simulink model "soar_unit_test"  (R2018b)
settings: Solver=FixedStepAuto  StartTime=0.0  StopTime=600  RelTol=1e-3
values from neighbouring files (symbols this model uses):
  hw0 = Jw * 0.10471975511966 * [ 1000; 1000; 1000 ]    [soar_unit_test_init.m]
  q0 = [ cosd(60/2); sind(60/2).*n ]    [soar_unit_test_init.m]
  qf = [ 1.0; 0.0; 0.0; 0.0 ]    [soar_unit_test_init.m]
  sI = [ 1.0; 0.0; 0.0 ]    [soar_unit_test_init.m]
  w0 = [ 0.0; 0.0; 0.0 ]    [soar_unit_test_init.m]
  wf = [ 0.0; 0.0; 0.0 ]    [soar_unit_test_init.m]
libraries: simulink x2, soar_lib x1
settings Model: Creator=Taylor  LastModifiedBy=Taylor
settings OptimizationCC: DefaultParameterBehavior=Inlined  UseDivisionForNetSlopeComputation=on  UseFloatMulNetSlope=on  InlineInvariantSignals=on  PassReuseOutputArgsAs=Individual arguments  ZeroExternalMemoryAtStartup=off  ZeroInternalMemoryAtStartup=off  NoFixptDivByZeroProtection=on  EfficientFloat2IntCast=on  LifeSpan=1
settings DebuggingCC: ParameterTunabilityLossMsg=error
settings HardwareCC: ProdBitPerPointer=32  ProdBitPerSizeT=32  ProdBitPerPtrDiffT=32  ProdLargestAtomicInteger=Long  ProdWordSize=32  ProdHWDeviceType=ARM Compatible->ARM 7
settings SFSimCC: SimUseLocalCustomCode=off  MATLABDynamicMemAlloc=off
settings RTWCC: SystemTargetFile=ert.tlc  TemplateMakefile=ert_default_tmf  GenerateReport=on  RTWUseLocalCustomCode=off  CustomInclude="\"/Users/Taylor/uw_cubesat_adcs/adcs/sw/components/adcs_oac/include/ecos/include\""  IncludeHyperlinkInReport=on  LaunchReport=on  GenerateTraceInfo=on  GenerateTraceReport=on  GenerateTraceReportSl=on  GenerateTraceReportSf=on  GenerateTraceReportEml=on  GenerateCodeMetricsReport=on
settings RTWCC: CustomSource=|
  | "/Users/Taylor/uw_cubesat_adcs/adcs/sw/components/adcs_oac/include/ecos/src/amd_1.c"
  | "/Users/Taylor/uw_cubesat_adcs/adcs/sw/components/adcs_oac/include/ecos/src/amd_2.c"
  | "/Users/Taylor/uw_cubesat_adcs/adcs/sw/components/adcs_oac/include/ecos/src/amd_aat.c"
  | "/Users/Taylor/uw_cubesat_adcs/adcs/sw/components/adcs_oac/include/ecos/src/amd_control.c"
  | "/Users/Taylor/uw_cubesat_adcs/adcs/sw/components/adcs_oac/include/ecos/src/amd_defaults.c"
  | "/Users/Taylor/uw_cubesat_adcs/adcs/sw/components/adcs_oac/include/ecos/src/amd_dump"
  | "/Users/Taylor/uw_cubesat_adcs/adcs/sw/components/adcs_oac/include/ecos/src/amd_global.c"
  | "/Users/Taylor/uw_cubesat_adcs/adcs/sw/components/adcs_oac/include/ecos/src/amd_info.c"
  | "/Users/Taylor/uw_cubesat_adcs/adcs/sw/components/adcs_oac/include/ecos/src/amd_order.c"
  | "/Users/Taylor/uw_cubesat_adcs/adcs/sw/components/adcs_oac/include/ecos/src/amd_post_tree.c"
  | "/Users/Taylor/uw_cubesat_adcs/adcs/sw/components/adcs_oac/include/ecos/src/amd_postorder.c"
  | "/Users/Taylor/uw_cubesat_adcs/adcs/sw/components/adcs_oac/include/ecos/src/amd_preprocess.c"
  | "/Users/Taylor/uw_cubesat_adcs/adcs/sw/components/adcs_oac/include/ecos/src/amd_valid.c"
  | "/Users/Taylor/uw_cubesat_adcs/adcs/sw/components/adcs_oac/include/ecos/src/cone.c"
  | "/Users/Taylor/uw_cubesat_adcs/adcs/sw/components/adcs_oac/include/ecos/src/ctrlc.c"
  | "/Users/Taylor/uw_cubesat_adcs/adcs/sw/components/adcs_oac/include/ecos/src/ecos.c"
  | "/Users/Taylor/uw_cubesat_adcs/adcs/sw/components/adcs_oac/include/ecos/src/equil.c"
  | "/Users/Taylor/uw_cubesat_adcs/adcs/sw/components/adcs_oac/include/ecos/src/expcone.c"
  | "/Users/Taylor/uw_cubesat_adcs/adcs/sw/components/adcs_oac/include/ecos/src/kkt.c"
  | "/Users/Taylor/uw_cubesat_adcs/adcs/sw/components/adcs_oac/include/ecos/src/ldl.c"
  | "/Users/Taylor/uw_cubesat_adcs/adcs/sw/components/adcs_oac/include/ecos/src/matlab_main.c"
  | "/Users/Taylor/uw_cubesat_adcs/adcs/sw/components/adcs_oac/include/ecos/src/preproc.c"
  | "/Users/Taylor/uw_cubesat_adcs/adcs/sw/components/adcs_oac/include/ecos/src/runecos.c"
  | "/Users/Taylor/uw_cubesat_adcs/adcs/sw/components/adcs_oac/include/ecos/src/spla.c"
  | "/Users/Taylor/uw_cubesat_adcs/adcs/sw/components/adcs_oac/include/ecos/src/splamm.c"
  | "/Users/Taylor/uw_cubesat_adcs/adcs/sw/components/adcs_oac/include/ecos/src/timer.c"
  | "/Users/Taylor/uw_cubesat_adcs/adcs/sw/components/adcs_oac/include/ecos/src/wright_omega.c"
settings CodeAppCC: ForceParamTrailComments=on  IgnoreCustomStorageClasses=off  OperatorAnnotations=on  SimulinkDataObjDesc=on  SFDataObjDesc=on  MATLABFcnDesc=on  CustomSymbolStrGlobalVar=rt$N$M  CustomSymbolStrType=$N$M  CustomSymbolStrFcn=$N$M$F  CustomSymbolStrMacro=$N$M  InsertBlockDesc=on  StateflowObjectComments=on  MATLABSourceComments=on
settings ERTTargetCC: TargetLangStandard=C99 (ISO)  MultiwordLength=2048  GenerateSampleERTMain=on  CombineSignalStateStructs=on  SupportAbsoluteTime=off  SupportComplex=off  SupportContinuousTime=on  SupportNonInlinedSFcns=on  InlinedParameterPlacement=NonHierarchical  ERTCustomFileTemplate=example_file_process.tlc  ERTFilePackagingFormat=CompactWithDataFile

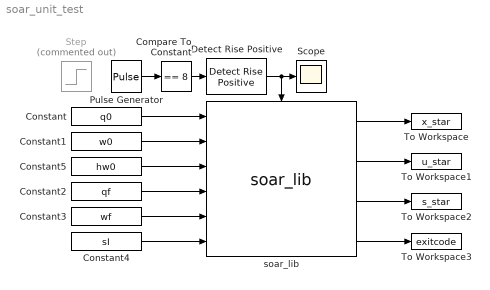
== system soar_unit_test ==
  Compare To Constant : simulink/Logic and Bit Operations/Compare To Constant  relop===  const=8  OutDataTypeStr=boolean
  Constant : Constant  Value=q0
  Constant1 : Constant  Value=w0
  Constant2 : Constant  Value=qf
  Constant3 : Constant  Value=wf
  Constant4 : Constant  Value=sI
  Constant5 : Constant  Value=hw0
  Detect Rise Positive : simulink/Logic and Bit Operations/Detect Rise Positive  vinit=0  OutDataTypeStr=boolean
  Pulse Generator : DiscretePulseGenerator  PulseType=Time based  Amplitude=8  Period=10  PulseWidth=50
  Scope : Scope
  Step : Step  Commented=on  Time=0  After=33  SampleTime=0
  To Workspace : ToWorkspace  VariableName=x_star  SampleTime=-1
  To Workspace1 : ToWorkspace  VariableName=u_star  SampleTime=-1
  To Workspace2 : ToWorkspace  VariableName=s_star  SampleTime=-1
  To Workspace3 : ToWorkspace  VariableName=exitcode  SampleTime=-1
  soar_lib : soar_lib/soar_lib  SystemSampleTime=-1
  wires:
  Constant/1 -> soar_lib/1
  Constant1/1 -> soar_lib/2
  Constant3/1 -> soar_lib/5
  Constant4/1 -> soar_lib/6
  soar_lib/1 -> To Workspace/1
  soar_lib/2 -> To Workspace1/1
  soar_lib/3 -> To Workspace2/1
  soar_lib/4 -> To Workspace3/1
  Pulse Generator/1 -> Compare To Constant/1
  Compare To Constant/1 -> Detect Rise Positive/1
  Detect Rise Positive/1 -> soar_lib/Trigger, Scope/1
  Constant5/1 -> soar_lib/3
  Constant2/1 -> soar_lib/4
